simulink model "NASY1"  (R2022b)
settings: Solver=FixedStepDiscrete  StartTime=0.0  StopTime=1000  RelTol=1e-3
PreLoadFcn:
  | eval([bdroot,'_init;'])
InitFcn:
  | eval([bdroot,'_init;'])
values from neighbouring files (symbols this model uses):
  bchannel = [0 0 0 1 -1/2 1/3 -1/4 1/5 -1/6 1/7]./10    [NASY1_init.m]
  Gupdate = 2^-9    (= 0.001953125)    [NASY1_init.m]
  Ntaps = 8    [NASY1_init.m]
libraries: simulink x3, hdlsllib x1
settings Model: Creator=Philipp  LastModifiedBy=Philipp

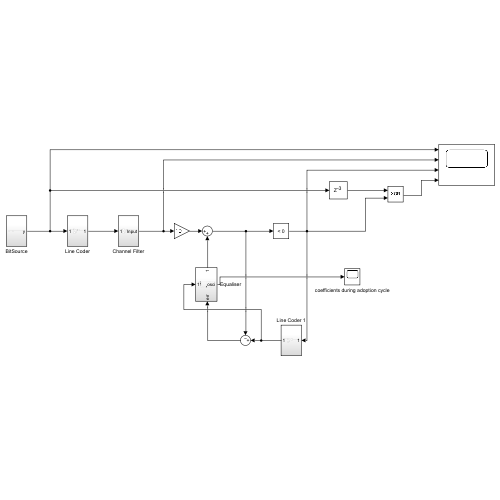
[thumbnail: Simulink's stored preview of the top-level diagram]
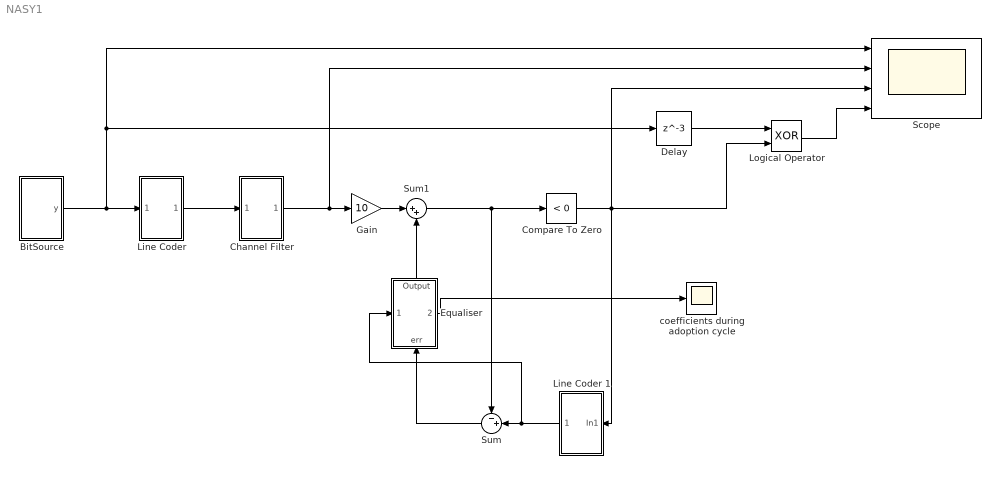
== system NASY1 ==
  BitSource : Subsystem
  Channel Filter : Subsystem
  Compare To Zero : hdlsllib/Logic and Bit Operations/Compare To Zero  relop=<  OutDataTypeStr=boolean
  Delay : Delay  DelayLength=3
  Equaliser : Subsystem
      settings: PortSchema="{\"entries\":[{\"content\":{\"sides\":[{\"content\":{\"connectorIds\":[\"In1\"]},\"type\":\"ConnectorPlacement.EquallySpacedRectSide\",\"uuid\":\"3a52bc40-cd0b-483c-b903-3ad34f040ca4\"},{\"content\":{\"connectorIds\":[\"Out1\"],\"side\":\"RIGHT\"},\"type\":\"ConnectorPlacement.EquallySpacedRectSide\",\"uuid\":\"ccc30700-4280-42a5-b749-6dd84debb21e\"},{\"content\":{\"connectorIds\":[\"In2\"],\"side\":\"TOP\"},\"type\":\"ConnectorPlacement.EquallySpacedRectSide\",\"uuid\":\"6189df6a-2e9b-42dd-9963-1eca64dfd213\"},{\"content\":{\"connectorIds\":[\"Out2\"],\"side\":\"BOTTOM\"},\"type\":\"ConnectorPlacement.EquallySpacedRectSide\",\"uuid\":\"72774d33-9e29-47b6-9d5a-2a56f8aff793\"}]},\"type\":\"ConnectorPlacement.EquallySpacedConnector\",\"uuid\":\"7a248eb0-7e33-44b4-8e09-7a6c6f38f4e1\"}],\"packageUris\":[\"http://schema.mathworks.com/mf0/Connector/R2020b\"],\"version\":\"1.0\"}"
  Gain : Gain  Gain=10
  Line Coder : Subsystem
  Line Coder 1 : Subsystem
  Logical Operator : Logic  Operator=XOR  AllPortsSameDT=off  OutDataTypeStr=boolean
  Scope : Scope  NumInputPorts=4
  Sum : Sum  Inputs=-+|
  Sum1 : Sum  Inputs=|++
  coefficients during adoption cycle : Scope
  wires:
  BitSource/1(y) -> Line Coder/1(In1), Scope/1, Delay/1
  Line Coder/1(Out1) -> Channel Filter/1(In1)
  Compare To Zero/1 -> Logical Operator/2, Line Coder 1/1(In1), Scope/3
  Delay/1 -> Logical Operator/1
  Logical Operator/1 -> Scope/4
  Channel Filter/1(Input) -> Scope/2, Gain/1
  Sum1/1 -> Sum/1, Compare To Zero/1
  Line Coder 1/1(1) -> Equaliser/2(1), Sum/2
  Sum/1 -> Equaliser/1(err)
  Equaliser/1(Output) -> Sum1/2
  Gain/1 -> Sum1/1
  Equaliser/2(osci) -> coefficients during adoption cycle/1

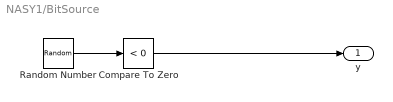
== system NASY1/BitSource ==
  Compare To Zero : simulink/Logic and Bit Operations/Compare To Zero  relop=<  OutDataTypeStr=boolean
  Random Number : RandomNumber  SampleTime=1
  y : Outport
  wires:
  Random Number/1 -> Compare To Zero/1
  Compare To Zero/1 -> y/1

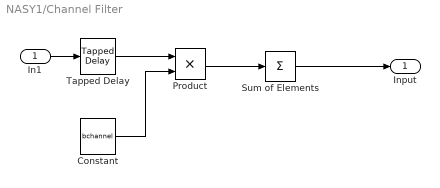
== system NASY1/Channel Filter ==
  In1 : Inport
  Constant : Constant  Value=bchannel
  Product : Product
  Sum of Elements : Sum  Inputs=+
  Tapped Delay : simulink/Discrete/Tapped Delay  vinit=0.0  samptime=-1  NumDelays=length(bchannel)-1  DelayOrder=Newest  includeCurrent=on
  Input : Outport
  wires:
  Constant/1 -> Product/2
  Tapped Delay/1 -> Product/1
  In1/1 -> Tapped Delay/1
  Product/1 -> Sum of Elements/1
  Sum of Elements/1 -> Input/1

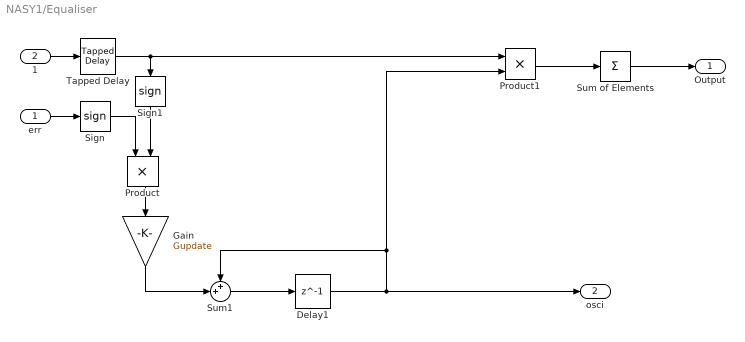
== system NASY1/Equaliser ==
  err : Inport
  1 : Inport  Port=2
  Delay1 : Delay  DelayLength=1
  Gain : Gain  Gain=Gupdate
  Product : Product
  Product1 : Product
  Sign : Signum
  Sign1 : Signum
  Sum of Elements : Sum  Inputs=+
  Sum1 : Sum  Inputs=++|
  Tapped Delay : simulink/Discrete/Tapped Delay  vinit=0  samptime=-1  NumDelays=Ntaps  DelayOrder=Newest  includeCurrent=off
  Output : Outport
  osci : Outport  Port=2
  wires:
  Product1/1 -> Sum of Elements/1
  Product/1 -> Gain/1
  Gain/1 -> Sum1/2
  Delay1/1 -> Product1/2, Sum1/1, osci/1
  Tapped Delay/1 -> Product1/1, Sign1/1
  err/1 -> Sign/1
  1/1 -> Tapped Delay/1
  Sum1/1 -> Delay1/1
  Sum of Elements/1 -> Output/1
  Sign/1 -> Product/1
  Sign1/1 -> Product/2

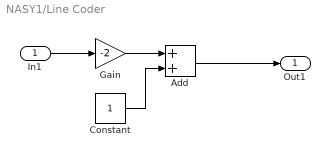
== system NASY1/Line Coder ==
  In1 : Inport
  Add : Sum
  Constant : Constant
  Gain : Gain  Gain=-2
  Out1 : Outport
  wires:
  Gain/1 -> Add/1
  Constant/1 -> Add/2
  In1/1 -> Gain/1
  Add/1 -> Out1/1

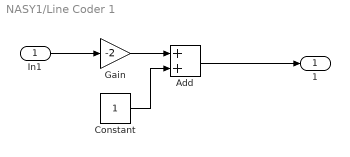
== system NASY1/Line Coder 1 ==
  In1 : Inport
  Add : Sum
  Constant : Constant
  Gain : Gain  Gain=-2
  1 : Outport
  wires:
  In1/1 -> Gain/1
  Constant/1 -> Add/2
  Add/1 -> 1/1
  Gain/1 -> Add/1
